simulink model "compliance_adjusting_controller_v4"  (R2020b)
settings: Solver=VariableStepAuto  StartTime=0.0  StopTime=40  RelTol=1e-3
values from neighbouring files (symbols this model uses):
  alpha = 0.001    [compliance_PLUS_energy_setup.m]    (also in compliance_adjusting_setup.m = 2; hyperbole_test.m = 1000)
  b0 = 2 * sqrt(k0 * m_R)    [compliance_PLUS_energy_setup.m]    (also in compliance_adjusting_setup.m = 2; energy_aware_setup.m = 20; optim_criteria.m = 0.2; plot_meshes.m = 0.2)
  C_max = 10    [compliance_PLUS_energy_setup.m]    (also in compliance_adjusting_setup.m = 0.2)
  F_cmax = 5    [compliance_PLUS_energy_setup.m]    (also in compliance_adjusting_setup.m)
  k0 = 20    [compliance_PLUS_energy_setup.m]    (also in compliance_adjusting_setup.m = 10; energy_aware_setup.m = 100; optim_criteria.m = 1; plot_meshes.m = 1)
  km = 100    [compliance_PLUS_energy_setup.m]    (also in compliance_adjusting_setup.m; energy_aware_setup.m; setup.m)
  m_R = 1    [compliance_PLUS_energy_setup.m]    (also in compliance_adjusting_setup.m; energy_aware_setup.m; setup.m)
  sigma = 0    [compliance_PLUS_energy_setup.m]    (also in compliance_adjusting_setup.m)
  T = 1/30    (= 0.0333333333333)    [compliance_PLUS_energy_setup.m]    (also in compliance_adjusting_setup.m)
  t_collision = 20    [compliance_PLUS_energy_setup.m]    (also in compliance_adjusting_setup.m; energy_aware_setup.m; setup.m)
  t_init = 2    [compliance_PLUS_energy_setup.m]    (also in compliance_adjusting_setup.m; energy_aware_setup.m; setup.m)
  x_O = 0.5    [compliance_PLUS_energy_setup.m]    (also in compliance_adjusting_setup.m; energy_aware_setup.m; setup.m)
  x_O2 = -2    [compliance_PLUS_energy_setup.m]    (also in compliance_adjusting_setup.m)
  x_R = 0    [compliance_PLUS_energy_setup.m]    (also in compliance_adjusting_setup.m; energy_aware_setup.m; setup.m)
libraries: neural x1
settings Model: Creator=kika  LastModifiedBy=kika

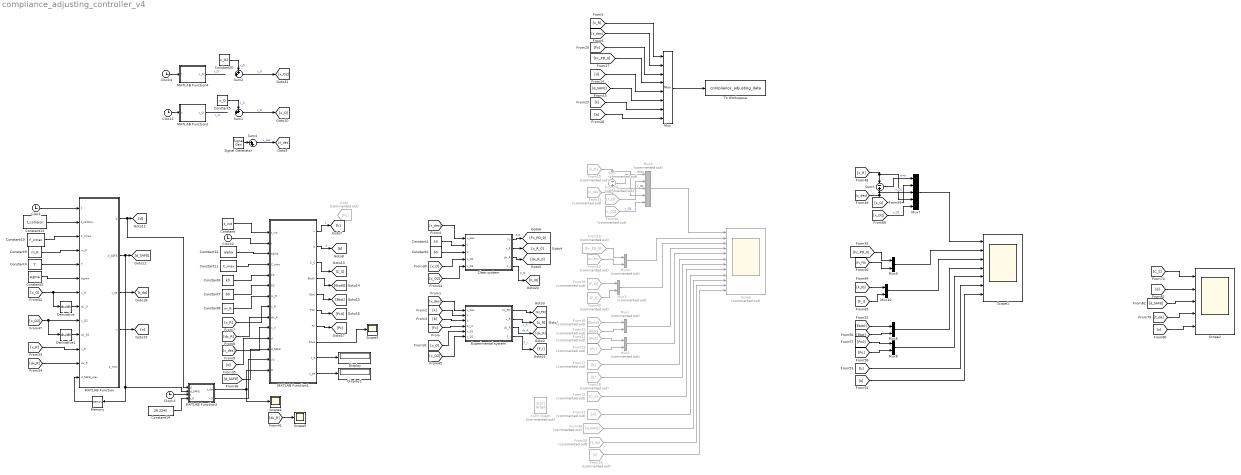
== system compliance_adjusting_controller_v4 ==
  Clear system : Subsystem
  Clock{,1..4} (5 alike) : Clock
  Constant : Constant  Value=t_init
  Constant1 : Constant  Value=k0
  Constant10 : Constant  Value=F_cmax
  Constant11 : Constant  Value=C_max
  Constant12 : Constant  Value=alpha
  Constant13 : Constant  Value=t_collision
  Constant14 : Constant  Value=26.2245
  Constant2 : Constant  Value=b0
  Constant20 : Constant  Value=x_O2
  Constant3 : Constant  Value=sigma
  Constant4 : Constant  Value=T
  Constant5 : Constant  Value=x_O
  Constant6 : Constant  Value=k0
  Constant7 : Constant  Value=b0
  Constant8 : Constant  Value=m_R
  Constant9 : Constant  Value=m_R
  Derivative : Derivative
  Derivative1 : Derivative
  Display : Display
  Display1 : Display
  Experimental system : Subsystem
  From10 : From  Commented=on  GotoTag=x_R
  From11 : From  Commented=on  GotoTag=x_des
  From12 : From  Commented=on  GotoTag=Fc_PD
  From13 : From  Commented=on  GotoTag=C_S
  From16 : From  Commented=on  GotoTag=Etot0
  From17 : From  Commented=on  GotoTag=k
  From18 : From  Commented=on  GotoTag=b
  From19 : From  Commented=on  GotoTag=Fc_PD_0
  From21 : From  Commented=on  GotoTag=Etot
  From22 : From  Commented=on  GotoTag=Pc0
  From23 : From  Commented=on  GotoTag=Pc
  From24 : From  Commented=on  GotoTag=x_O
  From28 : From  Commented=on  GotoTag=t_da
  From29 : From  Commented=on  GotoTag=n
  From37 : From  Commented=on  GotoTag=d
  From38 : From  Commented=on  GotoTag=d_SAFE
  From39 : From  Commented=on  GotoTag=F_I0
  From40 : From  Commented=on  GotoTag=F_I
  From46 : From  Commented=on  GotoTag=x_O2
  Goto : Goto  Commented=on  GotoTag=Fc
  MATLAB Function : MATLAB Function  TreatAsAtomicUnit=on
  MATLAB Function1 : MATLAB Function  TreatAsAtomicUnit=on
  MATLAB Function2 : MATLAB Function  TreatAsAtomicUnit=on
  MATLAB Function3 : MATLAB Function  TreatAsAtomicUnit=on
  MATLAB Function4 : MATLAB Function  TreatAsAtomicUnit=on
  Memory : Memory
  Mux : Mux  Inputs=8
  Mux{1,3..5} (4 alike) : Mux  Commented=on  Inputs=2
  Mux{6,8..10} (4 alike) : Mux  Inputs=2
  Mux2 : Mux  Commented=on  Inputs=5
  Mux7 : Mux  Inputs=5
  Scope : Scope  Commented=on  NumInputPorts=12
  Scope1 : Scope  NumInputPorts=7
  Scope2 : Scope  NumInputPorts=5
  Scope3 : Scope
  Scope4 : Scope
  Scope5 : Scope
  Signal Generator : SignalGenerator  Frequency=0.5  Units=rad/sec
  Sum : Sum  Commented=on  Inputs=-+
  Sum1 : Sum  Inputs=++|
  Sum2 : Sum  Inputs=++|
  Sum3 : Sum  Inputs=-+
  Sum4 : Sum  Inputs=|++
  To Workspace : ToWorkspace  VariableName=compliance_adjusting_data  SaveFormat=Timeseries  SampleTime=-1
  X(2Y) Graph : neural/Control Systems/X(2Y)  Graph  Commented=on  xmin=0  xmax=5  ymin=21  ymax=22  st=-1
      settings: SourceProductBaseCode=NN
  wires:
  Constant7/1 -> MATLAB Function1/6(b0)
  MATLAB Function1/1(k) -> [k]  "k"
  Constant8/1 -> MATLAB Function1/7(m_R)
  Constant6/1 -> MATLAB Function1/5(k0)
  Clock2/1 -> MATLAB Function1/2(t)
  MATLAB Function1/2(b) -> [b]  "b"
  Signal Generator/1 -> Sum4/1
  Constant/1 -> MATLAB Function1/1(t_init)
  [Fc] -> Experimental system/4(Fc_in)
  [x_des] -> Experimental system/1(x_des)
  Experimental system/2(x_R) -> [x_R]  "x_R"
  Experimental system/3(dx_R) -> [dx_R]  "dx_R"
  Experimental system/1(Fc_PD) -> [Fc_PD]
  Clear system/1(Fc) -> [Fc_PD_0]  "Fc0"
  Clear system/2(x_R) -> [x_R_0]
  Clear system/3(dx_R) -> [dx_R_0]
  [k] -> Experimental system/2(k)
  [b] -> Experimental system/3(b)
  [x_des] -> Clear system/1(x_des)
  Constant1/1 -> Clear system/2(k)
  Constant2/1 -> Clear system/3(b)
  [dx_R] -> MATLAB Function1/9(dx_R)
  [x_R] -> MATLAB Function1/8(x_R)
  Sum4/1 -> [x_des]  "x_des"
  [x_des] -> MATLAB Function1/10(x_V)
  From10/1 -> Mux2/4, Sum/1
  From11/1 -> Mux2/3, Sum/2
  Mux2/1 -> Scope/1
  From12/1 -> Mux4/2
  From17/1 -> Scope/6
  From18/1 -> Scope/7
  From19/1 -> Mux4/1
  Mux4/1 -> Scope/2
  Sum/1 -> Mux2/1  "error"
  Mux/1 -> To Workspace/1
  [x_O] -> Experimental system/5(x_O1)
  [x_O] -> Clear system/4(x_O1)
  [x_O] -> Derivative/1, MATLAB Function/7(x_O)
  [x_R] -> MATLAB Function/11(x_R)
  [dx_R] -> MATLAB Function/12(dx_R)
  Derivative/1 -> MATLAB Function/8(dx_O)
  Constant3/1 -> MATLAB Function/6(sigma)
  Constant4/1 -> MATLAB Function/5(T)
  Constant9/1 -> MATLAB Function/4(m_R)
  Constant10/1 -> MATLAB Function/3(F_cmax)
  Constant11/1 -> MATLAB Function1/4(C_max)
  Constant12/1 -> MATLAB Function1/3(alpha)
  [d_SAFE] -> MATLAB Function1/12(d_SAFE)
  [d] -> MATLAB Function1/11(d)
  MATLAB Function/1(d) -> MATLAB Function3/1(d), [d]
  MATLAB Function/2(d_SAFE) -> Memory/1, MATLAB Function3/2(d_SAFE), [d_SAFE]
  Constant13/1 -> MATLAB Function/2(t_collition)
  Clock/1 -> MATLAB Function/1(t)
  MATLAB Function1/3(C_S) -> [C_S]
  From13/1 -> Scope/8
  [d_SAFE] -> Mux/6
  [Fc_PD_0] -> Mux/4
  [d] -> Mux/5
  [k] -> Mux/7
  [b] -> Mux/8
  [Fc] -> Mux/3
  [x_des] -> Mux/2
  [x_R] -> Mux/1
  From37/1 -> Scope/9
  From38/1 -> Scope/10
  Mux1/1 -> Scope/4
  Mux3/1 -> Scope/5
  MATLAB Function1/7(Pc) -> [Pc]
  MATLAB Function1/6(Pc0) -> [Pc0]
  MATLAB Function1/5(Etot) -> [Etot]
  MATLAB Function1/4(Etot0) -> [Etot0]
  From16/1 -> Mux1/1
  From21/1 -> Mux1/2
  From22/1 -> Mux3/1
  From23/1 -> Mux3/2
  Constant5/1 -> Sum1/1  "x_O"
  From24/1 -> Mux2/2  "x_O1"
  Sum1/1 -> [x_O]  "x_O"
  MATLAB Function2/1(x_O) -> ?  "x_O"
  Clock1/1 -> MATLAB Function2/1(t)
  Memory/1 -> MATLAB Function/13(d_SAFE_prev)
  MATLAB Function/3(t_da) -> [t_da]
  MATLAB Function/4(n) -> [n]
  From28/1 -> Scope/11
  From29/1 -> Scope/12
  Clear system/4(F_I) -> [F_I0]  "F_I0"
  Experimental system/4(F_I) -> [F_I]  "F_I"
  From39/1 -> Mux5/1
  From40/1 -> Mux5/2
  Mux5/1 -> Scope/3
  [x_O2] -> Clear system/5(x_O2)
  [x_O2] -> Experimental system/6(x_O2)
  Constant20/1 -> Sum2/1  "x_O"
  MATLAB Function4/1(x_O) -> ?  "x_O"
  Sum2/1 -> [x_O2]  "x_O"
  Clock4/1 -> MATLAB Function4/1(t)
  From46/1 -> Mux2/5  "x_O2"
  [x_O2] -> Derivative1/1, MATLAB Function/9(x_O2)
  Derivative1/1 -> MATLAB Function/10(dx_O2)
  [Etot0] -> Mux6/1
  Mux8/1 -> Scope1/5
  Mux9/1 -> Scope1/2
  Mux7/1 -> Scope1/1
  [Pc] -> Mux8/2
  Sum3/1 -> Mux7/1  "error"
  Mux10/1 -> Scope1/3
  [Etot] -> Mux6/2
  [Fc_PD_0] -> Mux9/1
  [F_I0] -> Mux10/1
  [x_O2] -> Mux7/5  "x_O2"
  [Pc0] -> Mux8/1
  [x_R] -> Mux7/4, Sum3/1
  [F_I] -> Mux10/2
  [k] -> Scope1/6
  [Fc_PD] -> Mux9/2
  Mux6/1 -> Scope1/4
  [x_O] -> Mux7/2  "x_O1"
  [x_des] -> Mux7/3, Sum3/2
  [b] -> Scope1/7
  [C_S] -> Scope2/1
  [d] -> Scope2/2
  [d_SAFE] -> Scope2/3
  [t_da] -> Scope2/4
  [n] -> Scope2/5
  MATLAB Function1/8(Fdes) -> Scope3/1
  Clock3/1 -> MATLAB Function3/3(t)
  MATLAB Function3/1(t_da) -> Scope4/1, MATLAB Function1/14(tt)
  Constant14/1 -> MATLAB Function3/4(t_0)
  [dx_R] -> Scope5/1
  MATLAB Function3/2(v0) -> MATLAB Function1/13(v0)
  MATLAB Function1/9(t_a) -> Display/1
  MATLAB Function1/10(t_da) -> Display1/1

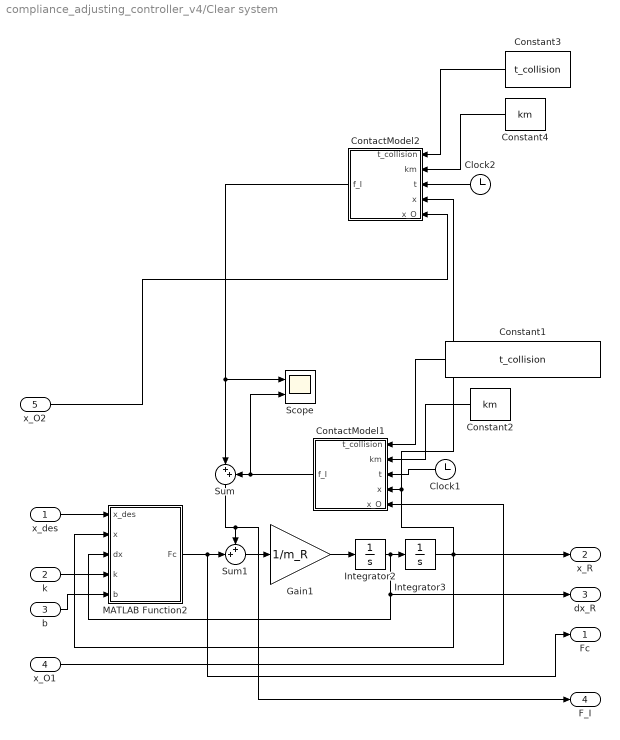
== system compliance_adjusting_controller_v4/Clear system ==
  x_des : Inport
  k : Inport  Port=2
  b : Inport  Port=3
  x_O1 : Inport  Port=4
  x_O2 : Inport  Port=5
  Clock1 : Clock
  Clock2 : Clock
  Constant1 : Constant  Value=t_collision
  Constant2 : Constant  Value=km
  Constant3 : Constant  Value=t_collision
  Constant4 : Constant  Value=km
  ContactModel1 : MATLAB Function  TreatAsAtomicUnit=on
  ContactModel2 : MATLAB Function  TreatAsAtomicUnit=on
  Gain1 : Gain  Gain=1/m_R
  Integrator2 : Integrator
  Integrator3 : Integrator  InitialCondition=x_R
  MATLAB Function2 : MATLAB Function  TreatAsAtomicUnit=on
  Scope : Scope  NumInputPorts=2
  Sum : Sum  Inputs=|++
  Sum1 : Sum  Inputs=++|
  Fc : Outport
  x_R : Outport  Port=2
  dx_R : Outport  Port=3
  F_I : Outport  Port=4
  wires:
  k/1 -> MATLAB Function2/4(k)
  ContactModel1/1(f_I) -> Scope/2, Sum/2
  Clock1/1 -> ContactModel1/3(t)
  x_des/1 -> MATLAB Function2/1(x_des)
  b/1 -> MATLAB Function2/5(b)
  Sum1/1 -> Gain1/1
  x_O1/1 -> ContactModel1/5(x_O)
  Gain1/1 -> Integrator2/1
  MATLAB Function2/1(Fc) -> Fc/1, Sum1/2
  Integrator2/1 -> dx_R/1, MATLAB Function2/3(dx), Integrator3/1
  Constant1/1 -> ContactModel1/1(t_collision)
  Constant2/1 -> ContactModel1/2(km)
  Constant3/1 -> ContactModel2/1(t_collision)
  Integrator3/1 -> x_R/1, ContactModel2/4(x), ContactModel1/4(x), MATLAB Function2/2(x)
  x_O2/1 -> ContactModel2/5(x_O)
  Constant4/1 -> ContactModel2/2(km)
  Clock2/1 -> ContactModel2/3(t)
  Sum/1 -> F_I/1, Sum1/1
  ContactModel2/1(f_I) -> Sum/1, Scope/1

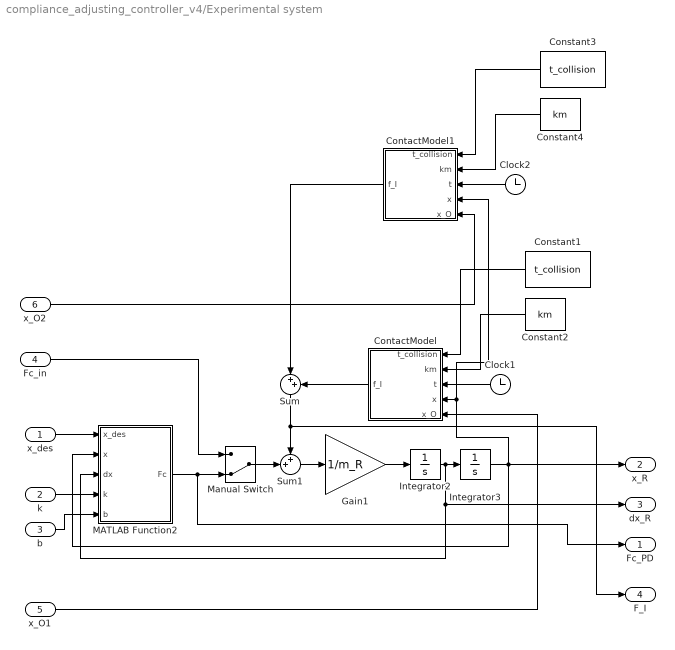
== system compliance_adjusting_controller_v4/Experimental system ==
  x_des : Inport
  k : Inport  Port=2
  b : Inport  Port=3
  Fc_in : Inport  Port=4
  x_O1 : Inport  Port=5
  x_O2 : Inport  Port=6
  Clock1 : Clock
  Clock2 : Clock
  Constant1 : Constant  Value=t_collision
  Constant2 : Constant  Value=km
  Constant3 : Constant  Value=t_collision
  Constant4 : Constant  Value=km
  ContactModel : MATLAB Function  TreatAsAtomicUnit=on
  ContactModel1 : MATLAB Function  TreatAsAtomicUnit=on
  Gain1 : Gain  Gain=1/m_R
  Integrator2 : Integrator
  Integrator3 : Integrator  InitialCondition=x_R
  MATLAB Function2 : MATLAB Function  TreatAsAtomicUnit=on
  Manual Switch : ManualSwitch  CurrentSetting=0
  Sum : Sum  Inputs=|++
  Sum1 : Sum  Inputs=++|
  Fc_PD : Outport
  x_R : Outport  Port=2
  dx_R : Outport  Port=3
  F_I : Outport  Port=4
  wires:
  k/1 -> MATLAB Function2/4(k)
  ContactModel/1(f_I) -> Sum/2
  Clock1/1 -> ContactModel/3(t)
  Integrator3/1 -> x_R/1, ContactModel1/4(x), ContactModel/4(x), MATLAB Function2/2(x)
  x_des/1 -> MATLAB Function2/1(x_des)
  b/1 -> MATLAB Function2/5(b)
  Sum1/1 -> Gain1/1
  x_O1/1 -> ContactModel/5(x_O)
  Gain1/1 -> Integrator2/1
  MATLAB Function2/1(Fc) -> Manual Switch/2, Fc_PD/1
  Integrator2/1 -> dx_R/1, MATLAB Function2/3(dx), Integrator3/1
  Constant1/1 -> ContactModel/1(t_collision)
  Constant2/1 -> ContactModel/2(km)
  Fc_in/1 -> Manual Switch/1
  Manual Switch/1 -> Sum1/2
  ContactModel1/1(f_I) -> Sum/1
  Constant4/1 -> ContactModel1/2(km)
  Constant3/1 -> ContactModel1/1(t_collision)
  Clock2/1 -> ContactModel1/3(t)
  x_O2/1 -> ContactModel1/5(x_O)
  Sum/1 -> F_I/1, Sum1/1

== matlab function compliance_adjusting_controller_v4/Clear system/ContactModel1 ==
  data: t_collision input; km input; t input; f_I output; x input; x_O input
function f_I = fcn(t_collision, km, t, x, x_O)


f_I = 0;

if t > t_collision
    if x > x_O
        f_I = km * (x_O - x);    
    end
end

% if t > t_collision
%     if abs(x) - abs(x_O) > 0
%         f_I = km * (abs(x_O) - abs(x));
%     end
% end

== matlab function compliance_adjusting_controller_v4/MATLAB Function ==
  data: t input; t_collition input; F_cmax input; m_R input; T input; sigma input; x_O input; dx_O input; x_O2 input; dx_O2 input; d output; x_R input; dx_R input; d_SAFE output; t_da output; n output; a_max output; d_SAFE_prev input
function [d, d_SAFE, t_da, n, a_max] = SENSING(t, t_collition, F_cmax, m_R, T, sigma, x_O, dx_O, x_O2, dx_O2, x_R, dx_R, d_SAFE_prev)

    
    d = 0.1;
    d_SAFE = 0;
    
    
    a_max = F_cmax / m_R;
    t_da1 = abs((dx_R - dx_O) / a_max);
    n1 = ceil(t_da1 / T);
    
    t_da2 = abs((dx_R - dx_O2) / a_max);
    n2 = ceil(t_da2 / T);
    
    t_da = 0;
    d1 = 0;
    d2 = 0;
    d_SAFE = 0;
    n = 0;
    if t > t_collition
        if x_R <= x_O
            d1 = abs(x_R - x_O);
            d1 = norm(x_R - x_O);
        else
            d1 = 0;
        end
        
        % d_SAFE calculation (deaceleration path length using F_cmax)
        d_SAFE1 = abs(dx_R - dx_O) * n1 * T;
%         d_SAFE = 0.4 * d_SAFE + 0.6 * d_SAFE_prev;
%         d_SAFE = 0.1;
    %     d_SAFE = abs(dx_R - dx_O) * n * T + 3 * sigma;
    
    
        if x_R >= x_O2
            d2 = abs(x_R - x_O2);
            d2 = norm(x_R - x_O2);
        else
            d2= 0;
        end
        
        % d_SAFE calculation (deaceleration path length using F_cmax)
        d_SAFE2 = abs(dx_R - dx_O2) * n2 * T;
        
        d_SAFE = d_SAFE1;
        d = d1;
        t_da = t_da1;
        n = n1;

        if d1 > d2 && d_SAFE > d_SAFE2
            d_SAFE = d_SAFE2;
            d = d2;
            t_da = t_da2;
            n = n2;
        end
        d_SAFE = 0.1
%          d_SAFE = 1.0 * d_SAFE;
%         if d_SAFE < 0.01
%             d_SAFE = 0.01;
%         end
%         if abs(dx_R)  < 0.000000001
%             d_SAFE = 0.000001;
%         end
    end

== matlab function compliance_adjusting_controller_v4/MATLAB Function2 ==
  data: t input; x_O output
function x_O = fcn(t)

    offset = -0.3;
    x_O = 1;
    if t > 23 && t < 35
        x_O = sin(0.5 * t + pi);
    end
    if t >= offset + 44.5 && t < offset +46.8
        x_O = 2*sin(1.5 * t - pi/6);
    end
    if t > 85
        x_O = 0.2;
    end

== matlab function compliance_adjusting_controller_v4/MATLAB Function3 ==
  data: d input; t_da output; d_SAFE input; t input; t_0 input; v0 output
function [t_da, v0]= fcn(d, d_SAFE, t, t_0)

    t_da = t;
    v0 = 0;
    if d < d_SAFE
        t_da = t - t_0;
        v0 = 0.544982;
    end

== matlab function compliance_adjusting_controller_v4/Experimental system/ContactModel1 ==
  data: t_collision input; km input; t input; f_I output; x input; x_O input
function f_I = fcn(t_collision, km, t, x, x_O)


f_I = 0;

if t > t_collision
    if x < x_O
        f_I = km * (x_O - x);
    end
end

== matlab function compliance_adjusting_controller_v4/Clear system/ContactModel2 ==
  data: t_collision input; km input; t input; f_I output; x input; x_O input
function f_I = fcn(t_collision, km, t, x, x_O)


f_I = 0;


if t > t_collision
    if x < x_O
        f_I = km * (x_O - x);
    end
end

== matlab function compliance_adjusting_controller_v4/MATLAB Function4 ==
  data: t input; x_O output
function x_O = fcn(t)

    x_O = 0;
    if t > 56 && t < 65
        x_O = sin(0.5 * t + pi) + 0.5;
    end
    if t > 71 && t < 85
        x_O = 1.5;
    end
%     if t >= 44.5 && t < 46.8
%         x_O = 3*sin(1.5 * t - pi/4);
%     end

== matlab function compliance_adjusting_controller_v4/Experimental system/ContactModel ==
  data: t_collision input; km input; t input; f_I output; x input; x_O input
function f_I = fcn(t_collision, km, t, x, x_O)


f_I = 0;

if t > t_collision
    if x > x_O
        f_I = km * (x_O - x);
    end
end

% if t > t_collision
%     if abs(x) - abs(x_O) > 0
%         f_I = km * (abs(x_O) - abs(x));
%     end
% end

== matlab function compliance_adjusting_controller_v4/Experimental system/MATLAB Function2 ==
  data: x_des input; Fc output; x input; dx input; k input; b input
function Fc = fcn(x_des, x, dx, k, b)

Fc = k * (x_des - x) - b * dx;

== matlab function compliance_adjusting_controller_v4/MATLAB Function1 ==
  data: t_init input; t input; alpha input; C_max input; k0 input; b0 input; m_R input; x_R input; k output; b output; dx_R input; x_V input; d input; d_SAFE input; C_S output; Etot0 output; Etot output; Pc0 output; Pc output; v0 input; Fdes output; tt input; t_a output; t_da output
function [k, b, C_S, Etot0, Etot, Pc0, Pc, Fdes, t_a, t_da] = compliance(t_init, t, alpha, C_max, k0, b0, m_R, x_R, dx_R, x_V, d, d_SAFE, v0, tt)

    Fdes = 0;
    a = 0;
    t_a = 0;
    t_da = 0;
    
    k = k0;
    b = b0;
    
    e = x_V - x_R;
    
    Etot0 = 0.5 * m_R * dx_R^2 + 0.5 * k * e^2;
    Pc0 = (k * e - b * dx_R) * dx_R;
    
    C_0 = 1 / k0;

    C_S = 0;
    if d <= d_SAFE
        D = (C_max * alpha * d)^2 + 4 * C_max * alpha * d_SAFE;
        beta = (-C_max * alpha * d + D) / (2 * C_max);
        gamma = - 1 / (alpha * d_SAFE + beta);
        
        C_S = 1 / (alpha * d + beta) + gamma;
    
        k = 1 / (C_0 + C_S);
%         if d < 0
%             k = 0
%         end
        % critical damping
%         b = 2 * sqrt(k * m_R);


        F_max = 5;
        a_max = F_max / m_R;
        j_max = 100000;

        t_a = a_max / j_max;
        t_da = v0 / a_max + t_a;

        a = 0;
        if tt <= t_a
            a = sign(v0) * j_max * tt;
        elseif tt <= (t_da - t_a)
            a = sign(v0) * a_max;
        elseif tt <= t_da
            a = sign(v0) * (j_max * t_da - j_max * tt);
        end
        
        if tt <= (t_da)
            a = sign(v0) * a_max;
        end
        
        Fdes = (m_R * a);
        
        b = abs((Fdes - k * (x_V - x_R)) / dx_R);
%         b = ((Fdes ) / dx_R);
        
    end
    
    Etot = 0.5 * m_R * dx_R^2 + 0.5 * k * e^2;
    Pc = (k * e - b * dx_R) * dx_R;

== matlab function compliance_adjusting_controller_v4/Clear system/MATLAB Function2 ==
  data: x_des input; Fc output; x input; dx input; k input; b input
function Fc = fcn(x_des, x, dx, k, b)

Fc = k * (x_des - x) - b * dx;
